simulink model "kopter_se_zavazim_state_feedback"  (R2024b)
(part 5 of 6)

0, 0, 0, 0, 0, 0, 0, 0, 0, 0, 0,                                                                                                                                                                                                                                                                                                                                                                                                                                                                                                                                                                                                                                                                                                                                                                                                                                                                                                                                                                                                                                                                                                                                                                                                  0,                                                                                                                                                                                                                                                                                                                                                                                                                                                                                                                                                                                                                                                                                                                                                                                                                                                                                                                                                                                                                                                                                                                                                                                                                                                                                                                                                                                                                                                                  0,                                                                                                                                                                                                                                                                                                                                                                                                                                                                                                                                                                                                                                                                                                                                                                                                                                                                                                                                                                                                                                                                                                                                                                                                        0, ((2*beta_dot_t*d*m*cos(alpha_t)*cos(beta_t) - alpha_dot_t*d*m*sin(alpha_t)*sin(beta_t))*(d^4*m^4*cos(beta_t)*sin(alpha_t)^4*sin(beta_t) - d^4*m^4*cos(beta_t)*sin(alpha_t)^2*sin(beta_t) - Ip*d^2*m^3*cos(beta_t)*sin(alpha_t)^2*sin(beta_t) - M*d^4*m^3*cos(beta_t)*sin(alpha_t)^2*sin(beta_t) + d^4*m^4*cos(alpha_t)^2*cos(beta_t)*sin(alpha_t)^2*sin(beta_t) + Ip*d^2*m^3*cos(alpha_t)^2*cos(beta_t)*sin(beta_t) + M*d^4*m^3*cos(alpha_t)^2*cos(beta_t)*sin(alpha_t)^2*sin(beta_t) + Ip*M*d^2*m^2*cos(alpha_t)^2*cos(beta_t)*sin(beta_t) - Ip*M*d^2*m^2*cos(beta_t)*sin(alpha_t)^2*sin(beta_t)))/(d^4*m^5*sin(alpha_t)^4 - Ip^2*m^3 - 3*Ip^2*M*m^2 - 3*Ip^2*M^2*m - d^4*m^5*sin(alpha_t)^2 - Ip^2*M^3 - Ip*d^2*m^4 + d^4*m^5*cos(beta_t)^2*sin(alpha_t)^2 - d^4*m^5*cos(beta_t)^2*sin(alpha_t)^4 + d^4*m^5*sin(alpha_t)^2*sin(beta_t)^2 - d^4*m^5*sin(alpha_t)^4*sin(beta_t)^2 - 3*M*d^4*m^4*sin(alpha_t)^2 + 2*M*d^4*m^4*sin(alpha_t)^4 - 3*Ip*M*d^2*m^3 - Ip*M^3*d^2*m - 3*M^2*d^4*m^3*sin(alpha_t)^2 - M^3*d^4*m^2*sin(alpha_t)^2 + M^2*d^4*m^3*sin(alpha_t)^4 - 3*Ip*M^2*d^2*m^2 + M^2*d^4*m^3*sin(alpha_t)^2*sin(beta_t)^2 - 2*Ip*M^2*d^2*m^2*sin(alpha_t)^2 + d^4*m^5*cos(alpha_t)^2*cos(beta_t)^2*sin(alpha_t)^2 - d^4*m^5*cos(alpha_t)^2*cos(beta_t)^4*sin(alpha_t)^2 + d^4*m^5*cos(alpha_t)^2*sin(alpha_t)^2*sin(beta_t)^2 - d^4*m^5*cos(alpha_t)^2*sin(alpha_t)^2*sin(beta_t)^4 + Ip*d^2*m^4*cos(alpha_t)^2*cos(beta_t)^2 + Ip*d^2*m^4*cos(alpha_t)^2*sin(beta_t)^2 + Ip*d^2*m^4*cos(beta_t)^2*sin(alpha_t)^2 + 2*M*d^4*m^4*cos(beta_t)^2*sin(alpha_t)^2 - M*d^4*m^4*cos(beta_t)^2*sin(alpha_t)^4 + Ip*d^2*m^4*sin(alpha_t)^2*sin(beta_t)^2 + 2*M*d^4*m^4*sin(alpha_t)^2*sin(beta_t)^2 - M*d^4*m^4*sin(alpha_t)^4*sin(beta_t)^2 - Ip*M*d^2*m^3*sin(alpha_t)^2 - Ip*M^3*d^2*m*sin(alpha_t)^2 + M^2*d^4*m^3*cos(beta_t)^2*sin(alpha_t)^2 + M^2*d^4*m^3*cos(alpha_t)^2*cos(beta_t)^2*sin(alpha_t)^2 + M^2*d^4*m^3*cos(alpha_t)^2*sin(alpha_t)^2*sin(beta_t)^2 + Ip*M^2*d^2*m^2*cos(alpha_t)^2*cos(beta_t)^2 + Ip*M^2*d^2*m^2*cos(alpha_t)^2*sin(beta_t)^2 + Ip*M^2*d^2*m^2*cos(beta_t)^2*sin(alpha_t)^2 + Ip*M^2*d^2*m^2*sin(alpha_t)^2*sin(beta_t)^2 - 2*d^4*m^5*cos(alpha_t)^2*cos(beta_t)^2*sin(alpha_t)^2*sin(beta_t)^2 + 2*M*d^4*m^4*cos(alpha_t)^2*cos(beta_t)^2*sin(alpha_t)^2 - M*d^4*m^4*cos(alpha_t)^2*cos(beta_t)^4*sin(alpha_t)^2 + 2*M*d^4*m^4*cos(alpha_t)^2*sin(alpha_t)^2*sin(beta_t)^2 - M*d^4*m^4*cos(alpha_t)^2*sin(alpha_t)^2*sin(beta_t)^4 + 2*Ip*M*d^2*m^3*cos(alpha_t)^2*cos(beta_t)^2 + 2*Ip*M*d^2*m^3*cos(alpha_t)^2*sin(beta_t)^2 + 2*Ip*M*d^2*m^3*cos(beta_t)^2*sin(alpha_t)^2 + 2*Ip*M*d^2*m^3*sin(alpha_t)^2*sin(beta_t)^2 - 2*M*d^4*m^4*cos(alpha_t)^2*cos(beta_t)^2*sin(alpha_t)^2*sin(beta_t)^2) - ((alpha_dot_t*d*m*cos(beta_t)*sin(alpha_t) + 2*beta_dot_t*d*m*cos(alpha_t)*sin(beta_t))*(Ip^2*M^2 + Ip^2*m^2 + d^4*m^4*sin(alpha_t)^2 - d^4*m^4*sin(alpha_t)^4 + Ip*d^2*m^3 + 2*Ip^2*M*m - d^4*m^4*cos(beta_t)^2*sin(alpha_t)^2 + d^4*m^4*cos(beta_t)^2*sin(alpha_t)^4 + 2*M*d^4*m^3*sin(alpha_t)^2 - M*d^4*m^3*sin(alpha_t)^4 + 2*Ip*M*d^2*m^2 + Ip*M^2*d^2*m + M^2*d^4*m^2*sin(alpha_t)^2 - d^4*m^4*cos(alpha_t)^2*sin(alpha_t)^2*sin(beta_t)^2 - Ip*d^2*m^3*cos(alpha_t)^2*sin(beta_t)^2 - Ip*d^2*m^3*cos(beta_t)^2*sin(alpha_t)^2 - M*d^4*m^3*cos(beta_t)^2*sin(alpha_t)^2 + Ip*M*d^2*m^2*sin(alpha_t)^2 + Ip*M^2*d^2*m*sin(alpha_t)^2 - M*d^4*m^3*cos(alpha_t)^2*sin(alpha_t)^2*sin(beta_t)^2 - Ip*M*d^2*m^2*cos(alpha_t)^2*sin(beta_t)^2 - Ip*M*d^2*m^2*cos(beta_t)^2*sin(alpha_t)^2))/(d^4*m^5*sin(alpha_t)^4 - Ip^2*m^3 - 3*Ip^2*M*m^2 - 3*Ip^2*M^2*m - d^4*m^5*sin(alpha_t)^2 - Ip^2*M^3 - Ip*d^2*m^4 + d^4*m^5*cos(beta_t)^2*sin(alpha_t)^2 - d^4*m^5*cos(beta_t)^2*sin(alpha_t)^4 + d^4*m^5*sin(alpha_t)^2*sin(beta_t)^2 - d^4*m^5*sin(alpha_t)^4*sin(beta_t)^2 - 3*M*d^4*m^4*sin(alpha_t)^2 + 2*M*d^4*m^4*sin(alpha_t)^4 - 3*Ip*M*d^2*m^3 - Ip*M^3*d^2*m - 3*M^2*d^4*m^3*sin(alpha_t)^2 - M^3*d^4*m^2*sin(alpha_t)^2 + M^2*d^4*m^3*sin(alpha_t)^4 - 3*Ip*M^2*d^2*m^2 + M^2*d^4*m^3*sin(alpha_t)^2*sin(beta_t)^2 - 2*Ip*M^2*d^2*m^2*sin(alpha_t)^2 + d^4*m^5*cos(alpha_t)^2*cos(beta_t)^2*sin(alpha_t)^2 - d^4*m^5*cos(alpha_t)^2*cos(beta_t)^4*sin(alpha_t)^2 + d^4*m^5*cos(alpha_t)^2*sin(alpha_t)^2*sin(beta_t)^2 - d^4*m^5*cos(alpha_t)^2*sin(alpha_t)^2*sin(beta_t)^4 + Ip*d^2*m^4*cos(alpha_t)^2*cos(beta_t)^2 + Ip*d^2*m^4*cos(alpha_t)^2*sin(beta_t)^2 + Ip*d^2*m^4*cos(beta_t)^2*sin(alpha_t)^2 + 2*M*d^4*m^4*cos(beta_t)^2*sin(alpha_t)^2 - M*d^4*m^4*cos(beta_t)^2*sin(alpha_t)^4 + Ip*d^2*m^4*sin(alpha_t)^2*sin(beta_t)^2 + 2*M*d^4*m^4*sin(alpha_t)^2*sin(beta_t)^2 - M*d^4*m^4*sin(alpha_t)^4*sin(beta_t)^2 - Ip*M*d^2*m^3*sin(alpha_t)^2 - Ip*M^3*d^2*m*sin(alpha_t)^2 + M^2*d^4*m^3*cos(beta_t)^2*sin(alpha_t)^2 + M^2*d^4*m^3*cos(alpha_t)^2*cos(beta_t)^2*sin(alpha_t)^2 + M^2*d^4*m^3*cos(alpha_t)^2*sin(alpha_t)^2*sin(beta_t)^2 + Ip*M^2*d^2*m^2*cos(alpha_t)^2*cos(beta_t)^2 + Ip*M^2*d^2*m^2*cos(alpha_t)^2*sin(beta_t)^2 + Ip*M^2*d^2*m^2*cos(beta_t)^2*sin(alpha_t)^2 + Ip*M^2*d^2*m^2*sin(alpha_t)^2*sin(beta_t)^2 - 2*d^4*m^5*cos(alpha_t)^2*cos(beta_t)^2*sin(alpha_t)^2*sin(beta_t)^2 + 2*M*d^4*m^4*cos(alpha_t)^2*cos(beta_t)^2*sin(alpha_t)^2 - M*d^4*m^4*cos(alpha_t)^2*cos(beta_t)^4*sin(alpha_t)^2 + 2*M*d^4*m^4*cos(alpha_t)^2*sin(alpha_t)^2*sin(beta_t)^2 - M*d^4*m^4*cos(alpha_t)^2*sin(alpha_t)^2*sin(beta_t)^4 + 2*Ip*M*d^2*m^3*cos(alpha_t)^2*cos(beta_t)^2 + 2*Ip*M*d^2*m^3*cos(alpha_t)^2*sin(beta_t)^2 + 2*Ip*M*d^2*m^3*cos(beta_t)^2*sin(alpha_t)^2 + 2*Ip*M*d^2*m^3*sin(alpha_t)^2*sin(beta_t)^2 - 2*M*d^4*m^4*cos(alpha_t)^2*cos(beta_t)^2*sin(alpha_t)^2*sin(beta_t)^2) - (alpha_dot_t*d*m*cos(alpha_t)*cos(beta_t)*(d^2*m*cos(alpha_t)*cos(beta_t)^2*sin(alpha_t) - d^2*m*cos(alpha_t)*sin(alpha_t) + d^2*m*cos(alpha_t)*sin(alpha_t)*sin(beta_t)^2))/(- d^2*m^2*cos(alpha_t)^2*cos(beta_t)^2 - d^2*m^2*cos(alpha_t)^2*sin(beta_t)^2 - d^2*m^2*sin(alpha_t)^2 + d^2*m^2 + M*d^2*m + Ip*m + Ip*M) - (alpha_dot_t*d^3*m^3*cos(alpha_t)^2*cos(beta_t)*sin(alpha_t))/(Ip*M^2 + Ip*m^2 + d^2*m^3 - d^2*m^3*sin(alpha_t)^2 + 2*M*d^2*m^2 + M^2*d^2*m + 2*Ip*M*m - d^2*m^3*cos(alpha_t)^2*cos(beta_t)^2 - d^2*m^3*cos(alpha_t)^2*sin(beta_t)^2 - M*d^2*m^2*sin(alpha_t)^2 - M*d^2*m^2*cos(alpha_t)^2*cos(beta_t)^2 - M*d^2*m^2*cos(alpha_t)^2*sin(beta_t)^2) - (beta_dot_t*d*m*sin(alpha_t)*sin(beta_t)*(2*d^2*m*cos(alpha_t)*cos(beta_t)^2*sin(alpha_t) + 2*d^2*m*cos(alpha_t)*sin(alpha_t)*sin(beta_t)^2))/(- d^2*m^2*cos(beta_t)^2*sin(alpha_t)^2 - d^2*m^2*sin(alpha_t)^2*sin(beta_t)^2 + d^2*m^2*sin(alpha_t)^2 + M*d^2*m*sin(alpha_t)^2 + Ip*m + Ip*M), - (beta_dot_t*d*m*cos(alpha_t)*cos(beta_t)*(m*cos(alpha_t)*sin(alpha_t)*d^2*cos(beta_t)^2 + m*cos(alpha_t)*sin(alpha_t)*d^2*sin(beta_t)^2))/(- d^2*m^2*cos(alpha_t)^2*cos(beta_t)^2 - d^2*m^2*cos(alpha_t)^2*sin(beta_t)^2 - d^2*m^2*sin(alpha_t)^2 + d^2*m^2 + M*d^2*m + Ip*m + Ip*M) - (beta_dot_t*d*m*sin(alpha_t)*sin(beta_t)*(d^4*m^4*cos(beta_t)*sin(alpha_t)^4*sin(beta_t) - d^4*m^4*cos(beta_t)*sin(alpha_t)^2*sin(beta_t) - Ip*d^2*m^3*cos(beta_t)*sin(alpha_t)^2*sin(beta_t) - M*d^4*m^3*cos(beta_t)*sin(alpha_t)^2*sin(beta_t) + d^4*m^4*cos(alpha_t)^2*cos(beta_t)*sin(alpha_t)^2*sin(beta_t) + Ip*d^2*m^3*cos(alpha_t)^2*cos(beta_t)*sin(beta_t) + M*d^4*m^3*cos(alpha_t)^2*cos(beta_t)*sin(alpha_t)^2*sin(beta_t) + Ip*M*d^2*m^2*cos(alpha_t)^2*cos(beta_t)*sin(beta_t) - Ip*M*d^2*m^2*cos(beta_t)*sin(alpha_t)^2*sin(beta_t)))/(d^4*m^5*sin(alpha_t)^4 - Ip^2*m^3 - 3*Ip^2*M*m^2 - 3*Ip^2*M^2*m - d^4*m^5*sin(alpha_t)^2 - Ip^2*M^3 - Ip*d^2*m^4 + d^4*m^5*cos(beta_t)^2*sin(alpha_t)^2 - d^4*m^5*cos(beta_t)^2*sin(alpha_t)^4 + d^4*m^5*sin(alpha_t)^2*sin(beta_t)^2 - d^4*m^5*sin(alpha_t)^4*sin(beta_t)^2 - 3*M*d^4*m^4*sin(alpha_t)^2 + 2*M*d^4*m^4*sin(alpha_t)^4 - 3*Ip*M*d^2*m^3 - Ip*M^3*d^2*m - 3*M^2*d^4*m^3*sin(alpha_t)^2 - M^3*d^4*m^2*sin(alpha_t)^2 + M^2*d^4*m^3*sin(alpha_t)^4 - 3*Ip*M^2*d^2*m^2 + M^2*d^4*m^3*sin(alpha_t)^2*sin(beta_t)^2 - 2*Ip*M^2*d^2*m^2*sin(alpha_t)^2 + d^4*m^5*cos(alpha_t)^2*cos(beta_t)^2*sin(alpha_t)^2 - d^4*m^5*cos(alpha_t)^2*cos(beta_t)^4*sin(alpha_t)^2 + d^4*m^5*cos(alpha_t)^2*sin(alpha_t)^2*sin(beta_t)^2 - d^4*m^5*cos(alpha_t)^2*sin(alpha_t)^2*sin(beta_t)^4 + Ip*d^2*m^4*cos(alpha_t)^2*cos(beta_t)^2 + Ip*d^2*m^4*cos(alpha_t)^2*sin(beta_t)^2 + Ip*d^2*m^4*cos(beta_t)^2*sin(alpha_t)^2 + 2*M*d^4*m^4*cos(beta_t)^2*sin(alpha_t)^2 - M*d^4*m^4*cos(beta_t)^2*sin(alpha_t)^4 + Ip*d^2*m^4*sin(alpha_t)^2*sin(beta_t)^2 + 2*M*d^4*m^4*sin(alpha_t)^2*sin(beta_t)^2 - M*d^4*m^4*sin(alpha_t)^4*sin(beta_t)^2 - Ip*M*d^2*m^3*sin(alpha_t)^2 - Ip*M^3*d^2*m*sin(alpha_t)^2 + M^2*d^4*m^3*cos(beta_t)^2*sin(alpha_t)^2 + M^2*d^4*m^3*cos(alpha_t)^2*cos(beta_t)^2*sin(alpha_t)^2 + M^2*d^4*m^3*cos(alpha_t)^2*sin(alpha_t)^2*sin(beta_t)^2 + Ip*M^2*d^2*m^2*cos(alpha_t)^2*cos(beta_t)^2 + Ip*M^2*d^2*m^2*cos(alpha_t)^2*sin(beta_t)^2 + Ip*M^2*d^2*m^2*cos(beta_t)^2*sin(alpha_t)^2 + Ip*M^2*d^2*m^2*sin(alpha_t)^2*sin(beta_t)^2 - 2*d^4*m^5*cos(alpha_t)^2*cos(beta_t)^2*sin(alpha_t)^2*sin(beta_t)^2 + 2*M*d^4*m^4*cos(alpha_t)^2*cos(beta_t)^2*sin(alpha_t)^2 - M*d^4*m^4*cos(alpha_t)^2*cos(beta_t)^4*sin(alpha_t)^2 + 2*M*d^4*m^4*cos(alpha_t)^2*sin(alpha_t)^2*sin(beta_t)^2 - M*d^4*m^4*cos(alpha_t)^2*sin(alpha_t)^2*sin(beta_t)^4 + 2*Ip*M*d^2*m^3*cos(alpha_t)^2*cos(beta_t)^2 + 2*Ip*M*d^2*m^3*cos(alpha_t)^2*sin(beta_t)^2 + 2*Ip*M*d^2*m^3*cos(beta_t)^2*sin(alpha_t)^2 + 2*Ip*M*d^2*m^3*sin(alpha_t)^2*sin(beta_t)^2 - 2*M*d^4*m^4*cos(alpha_t)^2*cos(beta_t)^2*sin(alpha_t)^2*sin(beta_t)^2) - (beta_dot_t*d*m*cos(beta_t)*sin(alpha_t)*(Ip^2*M^2 + Ip^2*m^2 + d^4*m^4*sin(alpha_t)^2 - d^4*m^4*sin(alpha_t)^4 + Ip*d^2*m^3 + 2*Ip^2*M*m - d^4*m^4*cos(beta_t)^2*sin(alpha_t)^2 + d^4*m^4*cos(beta_t)^2*sin(alpha_t)^4 + 2*M*d^4*m^3*sin(alpha_t)^2 - M*d^4*m^3*sin(alpha_t)^4 + 2*Ip*M*d^2*m^2 + Ip*M^2*d^2*m + M^2*d^4*m^2*sin(alpha_t)^2 - d^4*m^4*cos(alpha_t)^2*sin(alpha_t)^2*sin(beta_t)^2 - Ip*d^2*m^3*cos(alpha_t)^2*sin(beta_t)^2 - Ip*d^2*m^3*cos(beta_t)^2*sin(alpha_t)^2 - M*d^4*m^3*cos(beta_t)^2*sin(alpha_t)^2 + Ip*M*d^2*m^2*sin(alpha_t)^2 + Ip*M^2*d^2*m*sin(alpha_t)^2 - M*d^4*m^3*cos(alpha_t)^2*sin(alpha_t)^2*sin(beta_t)^2 - Ip*M*d^2*m^2*cos(alpha_t)^2*sin(beta_t)^2 - Ip*M*d^2*m^2*cos(beta_t)^2*sin(alpha_t)^2))/(d^4*m^5*sin(alpha_t)^4 - Ip^2*m^3 - 3*Ip^2*M*m^2 - 3*Ip^2*M^2*m - d^4*m^5*sin(alpha_t)^2 - Ip^2*M^3 - Ip*d^2*m^4 + d^4*m^5*cos(beta_t)^2*sin(alpha_t)^2 - d^4*m^5*cos(beta_t)^2*sin(alpha_t)^4 + d^4*m^5*sin(alpha_t)^2*sin(beta_t)^2 - d^4*m^5*sin(alpha_t)^4*sin(beta_t)^2 - 3*M*d^4*m^4*sin(alpha_t)^2 + 2*M*d^4*m^4*sin(alpha_t)^4 - 3*Ip*M*d^2*m^3 - Ip*M^3*d^2*m - 3*M^2*d^4*m^3*sin(alpha_t)^2 - M^3*d^4*m^2*sin(alpha_t)^2 + M^2*d^4*m^3*sin(alpha_t)^4 - 3*Ip*M^2*d^2*m^2 + M^2*d^4*m^3*sin(alpha_t)^2*sin(beta_t)^2 - 2*Ip*M^2*d^2*m^2*sin(alpha_t)^2 + d^4*m^5*cos(alpha_t)^2*cos(beta_t)^2*sin(alpha_t)^2 - d^4*m^5*cos(alpha_t)^2*cos(beta_t)^4*sin(alpha_t)^2 + d^4*m^5*cos(alpha_t)^2*sin(alpha_t)^2*sin(beta_t)^2 - d^4*m^5*cos(alpha_t)^2*sin(alpha_t)^2*sin(beta_t)^4 + Ip*d^2*m^4*cos(alpha_t)^2*cos(beta_t)^2 + Ip*d^2*m^4*cos(alpha_t)^2*sin(beta_t)^2 + Ip*d^2*m^4*cos(beta_t)^2*sin(alpha_t)^2 + 2*M*d^4*m^4*cos(beta_t)^2*sin(alpha_t)^2 - M*d^4*m^4*cos(beta_t)^2*sin(alpha_t)^4 + Ip*d^2*m^4*sin(alpha_t)^2*sin(beta_t)^2 + 2*M*d^4*m^4*sin(alpha_t)^2*sin(beta_t)^2 - M*d^4*m^4*sin(alpha_t)^4*sin(beta_t)^2 - Ip*M*d^2*m^3*sin(alpha_t)^2 - Ip*M^3*d^2*m*sin(alpha_t)^2 + M^2*d^4*m^3*cos(beta_t)^2*sin(alpha_t)^2 + M^2*d^4*m^3*cos(alpha_t)^2*cos(beta_t)^2*sin(alpha_t)^2 + M^2*d^4*m^3*cos(alpha_t)^2*sin(alpha_t)^2*sin(beta_t)^2 + Ip*M^2*d^2*m^2*cos(alpha_t)^2*cos(beta_t)^2 + Ip*M^2*d^2*m^2*cos(alpha_t)^2*sin(beta_t)^2 + Ip*M^2*d^2*m^2*cos(beta_t)^2*sin(alpha_t)^2 + Ip*M^2*d^2*m^2*sin(alpha_t)^2*sin(beta_t)^2 - 2*d^4*m^5*cos(alpha_t)^2*cos(beta_t)^2*sin(alpha_t)^2*sin(beta_t)^2 + 2*M*d^4*m^4*cos(alpha_t)^2*cos(beta_t)^2*sin(alpha_t)^2 - M*d^4*m^4*cos(alpha_t)^2*cos(beta_t)^4*sin(alpha_t)^2 + 2*M*d^4*m^4*cos(alpha_t)^2*sin(alpha_t)^2*sin(beta_t)^2 - M*d^4*m^4*cos(alpha_t)^2*sin(alpha_t)^2*sin(beta_t)^4 + 2*Ip*M*d^2*m^3*cos(alpha_t)^2*cos(beta_t)^2 + 2*Ip*M*d^2*m^3*cos(alpha_t)^2*sin(beta_t)^2 + 2*Ip*M*d^2*m^3*cos(beta_t)^2*sin(alpha_t)^2 + 2*Ip*M*d^2*m^3*sin(alpha_t)^2*sin(beta_t)^2 - 2*M*d^4*m^4*cos(alpha_t)^2*cos(beta_t)^2*sin(alpha_t)^2*sin(beta_t)^2);
0, 0, 0, 0, 0, 0, 0, 0, 0, 0, 0,                                                                                                                                                                                                                                                                                                                                                                                                                                                                                                                                                                                                                                                                                                                                                                                                                                                                                                                                                                                                                                                                                                                                                                                                  0,                                                                                                                                                                                                                                                                                                                                                                                                                                                                                                                                                                                                                                                                                                                                                                                                                                                                                                                                                                                                                                                                                                                                                                                                                                                                                                                                                                                                                                                                  0,                                                                                                                                                                                                                                                                                                                                                                                                                                                                                                                                                                                                                                                                                                                                                                                                                                                                                                                                                                                                                                                                                                                                                                                                        0, ((2*beta_dot_t*d*m*cos(alpha_t)*cos(beta_t) - alpha_dot_t*d*m*sin(alpha_t)*sin(beta_t))*(Ip^2*M^2 + Ip^2*m^2 + d^4*m^4*sin(alpha_t)^2 - d^4*m^4*sin(alpha_t)^4 + Ip*d^2*m^3 + 2*Ip^2*M*m - d^4*m^4*sin(alpha_t)^2*sin(beta_t)^2 + d^4*m^4*sin(alpha_t)^4*sin(beta_t)^2 + 2*M*d^4*m^3*sin(alpha_t)^2 - M*d^4*m^3*sin(alpha_t)^4 + 2*Ip*M*d^2*m^2 + Ip*M^2*d^2*m + M^2*d^4*m^2*sin(alpha_t)^2 - d^4*m^4*cos(alpha_t)^2*cos(beta_t)^2*sin(alpha_t)^2 - Ip*d^2*m^3*cos(alpha_t)^2*cos(beta_t)^2 - Ip*d^2*m^3*sin(alpha_t)^2*sin(beta_t)^2 - M*d^4*m^3*sin(alpha_t)^2*sin(beta_t)^2 + Ip*M*d^2*m^2*sin(alpha_t)^2 + Ip*M^2*d^2*m*sin(alpha_t)^2 - M*d^4*m^3*cos(alpha_t)^2*cos(beta_t)^2*sin(alpha_t)^2 - Ip*M*d^2*m^2*cos(alpha_t)^2*cos(beta_t)^2 - Ip*M*d^2*m^2*sin(alpha_t)^2*sin(beta_t)^2))/(d^4*m^5*sin(alpha_t)^4 - Ip^2*m^3 - 3*Ip^2*M*m^2 - 3*Ip^2*M^2*m - d^4*m^5*sin(alpha_t)^2 - Ip^2*M^3 - Ip*d^2*m^4 + d^4*m^5*cos(beta_t)^2*sin(alpha_t)^2 - d^4*m^5*cos(beta_t)^2*sin(alpha_t)^4 + d^4*m^5*sin(alpha_t)^2*sin(beta_t)^2 - d^4*m^5*sin(alpha_t)^4*sin(beta_t)^2 - 3*M*d^4*m^4*sin(alpha_t)^2 + 2*M*d^4*m^4*sin(alpha_t)^4 - 3*Ip*M*d^2*m^3 - Ip*M^3*d^2*m - 3*M^2*d^4*m^3*sin(alpha_t)^2 - M^3*d^4*m^2*sin(alpha_t)^2 + M^2*d^4*m^3*sin(alpha_t)^4 - 3*Ip*M^2*d^2*m^2 + M^2*d^4*m^3*sin(alpha_t)^2*sin(beta_t)^2 - 2*Ip*M^2*d^2*m^2*sin(alpha_t)^2 + d^4*m^5*cos(alpha_t)^2*cos(beta_t)^2*sin(alpha_t)^2 - d^4*m^5*cos(alpha_t)^2*cos(beta_t)^4*sin(alpha_t)^2 + d^4*m^5*cos(alpha_t)^2*sin(alpha_t)^2*sin(beta_t)^2 - d^4*m^5*cos(alpha_t)^2*sin(alpha_t)^2*sin(beta_t)^4 + Ip*d^2*m^4*cos(alpha_t)^2*cos(beta_t)^2 + Ip*d^2*m^4*cos(alpha_t)^2*sin(beta_t)^2 + Ip*d^2*m^4*cos(beta_t)^2*sin(alpha_t)^2 + 2*M*d^4*m^4*cos(beta_t)^2*sin(alpha_t)^2 - M*d^4*m^4*cos(beta_t)^2*sin(alpha_t)^4 + Ip*d^2*m^4*sin(alpha_t)^2*sin(beta_t)^2 + 2*M*d^4*m^4*sin(alpha_t)^2*sin(beta_t)^2 - M*d^4*m^4*sin(alpha_t)^4*sin(beta_t)^2 - Ip*M*d^2*m^3*sin(alpha_t)^2 - Ip*M^3*d^2*m*sin(alpha_t)^2 + M^2*d^4*m^3*cos(beta_t)^2*sin(alpha_t)^2 + M^2*d^4*m^3*cos(alpha_t)^2*cos(beta_t)^2*sin(alpha_t)^2 + M^2*d^4*m^3*cos(alpha_t)^2*sin(alpha_t)^2*sin(beta_t)^2 + Ip*M^2*d^2*m^2*cos(alpha_t)^2*cos(beta_t)^2 + Ip*M^2*d^2*m^2*cos(alpha_t)^2*sin(beta_t)^2 + Ip*M^2*d^2*m^2*cos(beta_t)^2*sin(alpha_t)^2 + Ip*M^2*d^2*m^2*sin(alpha_t)^2*sin(beta_t)^2 - 2*d^4*m^5*cos(alpha_t)^2*cos(beta_t)^2*sin(alpha_t)^2*sin(beta_t)^2 + 2*M*d^4*m^4*cos(alpha_t)^2*cos(beta_t)^2*sin(alpha_t)^2 - M*d^4*m^4*cos(alpha_t)^2*cos(beta_t)^4*sin(alpha_t)^2 + 2*M*d^4*m^4*cos(alpha_t)^2*sin(alpha_t)^2*sin(beta_t)^2 - M*d^4*m^4*cos(alpha_t)^2*sin(alpha_t)^2*sin(beta_t)^4 + 2*Ip*M*d^2*m^3*cos(alpha_t)^2*cos(beta_t)^2 + 2*Ip*M*d^2*m^3*cos(alpha_t)^2*sin(beta_t)^2 + 2*Ip*M*d^2*m^3*cos(beta_t)^2*sin(alpha_t)^2 + 2*Ip*M*d^2*m^3*sin(alpha_t)^2*sin(beta_t)^2 - 2*M*d^4*m^4*cos(alpha_t)^2*cos(beta_t)^2*sin(alpha_t)^2*sin(beta_t)^2) - ((alpha_dot_t*d*m*cos(beta_t)*sin(alpha_t) + 2*beta_dot_t*d*m*cos(alpha_t)*sin(beta_t))*(d^4*m^4*cos(beta_t)*sin(alpha_t)^4*sin(beta_t) - d^4*m^4*cos(beta_t)*sin(alpha_t)^2*sin(beta_t) - Ip*d^2*m^3*cos(beta_t)*sin(alpha_t)^2*sin(beta_t) - M*d^4*m^3*cos(beta_t)*sin(alpha_t)^2*sin(beta_t) + d^4*m^4*cos(alpha_t)^2*cos(beta_t)*sin(alpha_t)^2*sin(beta_t) + Ip*d^2*m^3*cos(alpha_t)^2*cos(beta_t)*sin(beta_t) + M*d^4*m^3*cos(alpha_t)^2*cos(beta_t)*sin(alpha_t)^2*sin(beta_t) + Ip*M*d^2*m^2*cos(alpha_t)^2*cos(beta_t)*sin(beta_t) - Ip*M*d^2*m^2*cos(beta_t)*sin(alpha_t)^2*sin(beta_t)))/(d^4*m^5*sin(alpha_t)^4 - Ip^2*m^3 - 3*Ip^2*M*m^2 - 3*Ip^2*M^2*m - d^4*m^5*sin(alpha_t)^2 - Ip^2*M^3 - Ip*d^2*m^4 + d^4*m^5*cos(beta_t)^2*sin(alpha_t)^2 - d^4*m^5*cos(beta_t)^2*sin(alpha_t)^4 + d^4*m^5*sin(alpha_t)^2*sin(beta_t)^2 - d^4*m^5*sin(alpha_t)^4*sin(beta_t)^2 - 3*M*d^4*m^4*sin(alpha_t)^2 + 2*M*d^4*m^4*sin(alpha_t)^4 - 3*Ip*M*d^2*m^3 - Ip*M^3*d^2*m - 3*M^2*d^4*m^3*sin(alpha_t)^2 - M^3*d^4*m^2*sin(alpha_t)^2 + M^2*d^4*m^3*sin(alpha_t)^4 - 3*Ip*M^2*d^2*m^2 + M^2*d^4*m^3*sin(alpha_t)^2*sin(beta_t)^2 - 2*Ip*M^2*d^2*m^2*sin(alpha_t)^2 + d^4*m^5*cos(alpha_t)^2*cos(beta_t)^2*sin(alpha_t)^2 - d^4*m^5*cos(alpha_t)^2*cos(beta_t)^4*sin(alpha_t)^2 + d^4*m^5*cos(alpha_t)^2*sin(alpha_t)^2*sin(beta_t)^2 - d^4*m^5*cos(alpha_t)^2*sin(alpha_t)^2*sin(beta_t)^4 + Ip*d^2*m^4*cos(alpha_t)^2*cos(beta_t)^2 + Ip*d^2*m^4*cos(alpha_t)^2*sin(beta_t)^2 + Ip*d^2*m^4*cos(beta_t)^2*sin(alpha_t)^2 + 2*M*d^4*m^4*cos(beta_t)^2*sin(alpha_t)^2 - M*d^4*m^4*cos(beta_t)^2*sin(alpha_t)^4 + Ip*d^2*m^4*sin(alpha_t)^2*sin(beta_t)^2 + 2*M*d^4*m^4*sin(alpha_t)^2*sin(beta_t)^2 - M*d^4*m^4*sin(alpha_t)^4*sin(beta_t)^2 - Ip*M*d^2*m^3*sin(alpha_t)^2 - Ip*M^3*d^2*m*sin(alpha_t)^2 + M^2*d^4*m^3*cos(beta_t)^2*sin(alpha_t)^2 + M^2*d^4*m^3*cos(alpha_t)^2*cos(beta_t)^2*sin(alpha_t)^2 + M^2*d^4*m^3*cos(alpha_t)^2*sin(alpha_t)^2*sin(beta_t)^2 + Ip*M^2*d^2*m^2*cos(alpha_t)^2*cos(beta_t)^2 + Ip*M^2*d^2*m^2*cos(alpha_t)^2*sin(beta_t)^2 + Ip*M^2*d^2*m^2*cos(beta_t)^2*sin(alpha_t)^2 + Ip*M^2*d^2*m^2*sin(alpha_t)^2*sin(beta_t)^2 - 2*d^4*m^5*cos(alpha_t)^2*cos(beta_t)^2*sin(alpha_t)^2*sin(beta_t)^2 + 2*M*d^4*m^4*cos(alpha_t)^2*cos(beta_t)^2*sin(alpha_t)^2 - M*d^4*m^4*cos(alpha_t)^2*cos(beta_t)^4*sin(alpha_t)^2 + 2*M*d^4*m^4*cos(alpha_t)^2*sin(alpha_t)^2*sin(beta_t)^2 - M*d^4*m^4*cos(alpha_t)^2*sin(alpha_t)^2*sin(beta_t)^4 + 2*Ip*M*d^2*m^3*cos(alpha_t)^2*cos(beta_t)^2 + 2*Ip*M*d^2*m^3*cos(alpha_t)^2*sin(beta_t)^2 + 2*Ip*M*d^2*m^3*cos(beta_t)^2*sin(alpha_t)^2 + 2*Ip*M*d^2*m^3*sin(alpha_t)^2*sin(beta_t)^2 - 2*M*d^4*m^4*cos(alpha_t)^2*cos(beta_t)^2*sin(alpha_t)^2*sin(beta_t)^2) - (alpha_dot_t*d*m*cos(alpha_t)*sin(beta_t)*(d^2*m*cos(alpha_t)*cos(beta_t)^2*sin(alpha_t) - d^2*m*cos(alpha_t)*sin(alpha_t) + d^2*m*cos(alpha_t)*sin(alpha_t)*sin(beta_t)^2))/(- d^2*m^2*cos(alpha_t)^2*cos(beta_t)^2 - d^2*m^2*cos(alpha_t)^2*sin(beta_t)^2 - d^2*m^2*sin(alpha_t)^2 + d^2*m^2 + M*d^2*m + Ip*m + Ip*M) - (alpha_dot_t*d^3*m^3*cos(alpha_t)^2*sin(alpha_t)*sin(beta_t))/(Ip*M^2 + Ip*m^2 + d^2*m^3 - d^2*m^3*sin(alpha_t)^2 + 2*M*d^2*m^2 + M^2*d^2*m + 2*Ip*M*m - d^2*m^3*cos(alpha_t)^2*cos(beta_t)^2 - d^2*m^3*cos(alpha_t)^2*sin(beta_t)^2 - M*d^2*m^2*sin(alpha_t)^2 - M*d^2*m^2*cos(alpha_t)^2*cos(beta_t)^2 - M*d^2*m^2*cos(alpha_t)^2*sin(beta_t)^2) + (beta_dot_t*d*m*cos(beta_t)*sin(alpha_t)*(2*d^2*m*cos(alpha_t)*cos(beta_t)^2*sin(alpha_t) + 2*d^2*m*cos(alpha_t)*sin(alpha_t)*sin(beta_t)^2))/(- d^2*m^2*cos(beta_t)^2*sin(alpha_t)^2 - d^2*m^2*sin(alpha_t)^2*sin(beta_t)^2 + d^2*m^2*sin(alpha_t)^2 + M*d^2*m*sin(alpha_t)^2 + Ip*m + Ip*M), - (beta_dot_t*d*m*cos(alpha_t)*sin(beta_t)*(m*cos(alpha_t)*sin(alpha_t)*d^2*cos(beta_t)^2 + m*cos(alpha_t)*sin(alpha_t)*d^2*sin(beta_t)^2))/(- d^2*m^2*cos(alpha_t)^2*cos(beta_t)^2 - d^2*m^2*cos(alpha_t)^2*sin(beta_t)^2 - d^2*m^2*sin(alpha_t)^2 + d^2*m^2 + M*d^2*m + Ip*m + Ip*M) - (beta_dot_t*d*m*cos(beta_t)*sin(alpha_t)*(d^4*m^4*cos(beta_t)*sin(alpha_t)^4*sin(beta_t) - d^4*m^4*cos(beta_t)*sin(alpha_t)^2*sin(beta_t) - Ip*d^2*m^3*cos(beta_t)*sin(alpha_t)^2*sin(beta_t) - M*d^4*m^3*cos(beta_t)*sin(alpha_t)^2*sin(beta_t) + d^4*m^4*cos(alpha_t)^2*cos(beta_t)*sin(alpha_t)^2*sin(beta_t) + Ip*d^2*m^3*cos(alpha_t)^2*cos(beta_t)*sin(beta_t) + M*d^4*m^3*cos(alpha_t)^2*cos(beta_t)*sin(alpha_t)^2*sin(beta_t) + Ip*M*d^2*m^2*cos(alpha_t)^2*cos(beta_t)*sin(beta_t) - Ip*M*d^2*m^2*cos(beta_t)*sin(alpha_t)^2*sin(beta_t)))/(d^4*m^5*sin(alpha_t)^4 - Ip^2*m^3 - 3*Ip^2*M*m^2 - 3*Ip^2*M^2*m - d^4*m^5*sin(alpha_t)^2 - Ip^2*M^3 - Ip*d^2*m^4 + d^4*m^5*cos(beta_t)^2*sin(alpha_t)^2 - d^4*m^5*cos(beta_t)^2*sin(alpha_t)^4 + d^4*m^5*sin(alpha_t)^2*sin(beta_t)^2 - d^4*m^5*sin(alpha_t)^4*sin(beta_t)^2 - 3*M*d^4*m^4*sin(alpha_t)^2 + 2*M*d^4*m^4*sin(alpha_t)^4 - 3*Ip*M*d^2*m^3 - Ip*M^3*d^2*m - 3*M^2*d^4*m^3*sin(alpha_t)^2 - M^3*d^4*m^2*sin(alpha_t)^2 + M^2*d^4*m^3*sin(alpha_t)^4 - 3*Ip*M^2*d^2*m^2 + M^2*d^4*m^3*sin(alpha_t)^2*sin(beta_t)^2 - 2*Ip*M^2*d^2*m^2*sin(alpha_t)^2 + d^4*m^5*cos(alpha_t)^2*cos(beta_t)^2*sin(alpha_t)^2 - d^4*m^5*cos(alpha_t)^2*cos(beta_t)^4*sin(alpha_t)^2 + d^4*m^5*cos(alpha_t)^2*sin(alpha_t)^2*sin(beta_t)^2 - d^4*m^5*cos(alpha_t)^2*sin(alpha_t)^2*sin(beta_t)^4 + Ip*d^2*m^4*cos(alpha_t)^2*cos(beta_t)^2 + Ip*d^2*m^4*cos(alpha_t)^2*sin(beta_t)^2 + Ip*d^2*m^4*cos(beta_t)^2*sin(alpha_t)^2 + 2*M*d^4*m^4*cos(beta_t)^2*sin(alpha_t)^2 - M*d^4*m^4*cos(beta_t)^2*sin(alpha_t)^4 + Ip*d^2*m^4*sin(alpha_t)^2*sin(beta_t)^2 + 2*M*d^4*m^4*sin(alpha_t)^2*sin(beta_t)^2 - M*d^4*m^4*sin(alpha_t)^4*sin(beta_t)^2 - Ip*M*d^2*m^3*sin(alpha_t)^2 - Ip*M^3*d^2*m*sin(alpha_t)^2 + M^2*d^4*m^3*cos(beta_t)^2*sin(alpha_t)^2 + M^2*d^4*m^3*cos(alpha_t)^2*cos(beta_t)^2*sin(alpha_t)^2 + M^2*d^4*m^3*cos(alpha_t)^2*sin(alpha_t)^2*sin(beta_t)^2 + Ip*M^2*d^2*m^2*cos(alpha_t)^2*cos(beta_t)^2 + Ip*M^2*d^2*m^2*cos(alpha_t)^2*sin(beta_t)^2 + Ip*M^2*d^2*m^2*cos(beta_t)^2*sin(alpha_t)^2 + Ip*M^2*d^2*m^2*sin(alpha_t)^2*sin(beta_t)^2 - 2*d^4*m^5*cos(alpha_t)^2*cos(beta_t)^2*sin(alpha_t)^2*sin(beta_t)^2 + 2*M*d^4*m^4*cos(alpha_t)^2*cos(beta_t)^2*sin(alpha_t)^2 - M*d^4*m^4*cos(alpha_t)^2*cos(beta_t)^4*sin(alpha_t)^2 + 2*M*d^4*m^4*cos(alpha_t)^2*sin(alpha_t)^2*sin(beta_t)^2 - M*d^4*m^4*cos(alpha_t)^2*sin(alpha_t)^2*sin(beta_t)^4 + 2*Ip*M*d^2*m^3*cos(alpha_t)^2*cos(beta_t)^2 + 2*Ip*M*d^2*m^3*cos(alpha_t)^2*sin(beta_t)^2 + 2*Ip*M*d^2*m^3*cos(beta_t)^2*sin(alpha_t)^2 + 2*Ip*M*d^2*m^3*sin(alpha_t)^2*sin(beta_t)^2 - 2*M*d^4*m^4*cos(alpha_t)^2*cos(beta_t)^2*sin(alpha_t)^2*sin(beta_t)^2) - (beta_dot_t*d*m*sin(alpha_t)*sin(beta_t)*(Ip^2*M^2 + Ip^2*m^2 + d^4*m^4*sin(alpha_t)^2 - d^4*m^4*sin(alpha_t)^4 + Ip*d^2*m^3 + 2*Ip^2*M*m - d^4*m^4*sin(alpha_t)^2*sin(beta_t)^2 + d^4*m^4*sin(alpha_t)^4*sin(beta_t)^2 + 2*M*d^4*m^3*sin(alpha_t)^2 - M*d^4*m^3*sin(alpha_t)^4 + 2*Ip*M*d^2*m^2 + Ip*M^2*d^2*m + M^2*d^4*m^2*sin(alpha_t)^2 - d^4*m^4*cos(alpha_t)^2*cos(beta_t)^2*sin(alpha_t)^2 - Ip*d^2*m^3*cos(alpha_t)^2*cos(beta_t)^2 - Ip*d^2*m^3*sin(alpha_t)^2*sin(beta_t)^2 - M*d^4*m^3*sin(alpha_t)^2*sin(beta_t)^2 + Ip*M*d^2*m^2*sin(alpha_t)^2 + Ip*M^2*d^2*m*sin(alpha_t)^2 - M*d^4*m^3*cos(alpha_t)^2*cos(beta_t)^2*sin(alpha_t)^2 - Ip*M*d^2*m^2*cos(alpha_t)^2*cos(beta_t)^2 - Ip*M*d^2*m^2*sin(alpha_t)^2*sin(beta_t)^2))/(d^4*m^5*sin(alpha_t)^4 - Ip^2*m^3 - 3*Ip^2*M*m^2 - 3*Ip^2*M^2*m - d^4*m^5*sin(alpha_t)^2 - Ip^2*M^3 - Ip*d^2*m^4 + d^4*m^5*cos(beta_t)^2*sin(alpha_t)^2 - d^4*m^5*cos(beta_t)^2*sin(alpha_t)^4 + d^4*m^5*sin(alpha_t)^2*sin(beta_t)^2 - d^4*m^5*sin(alpha_t)^4*sin(beta_t)^2 - 3*M*d^4*m^4*sin(alpha_t)^2 + 2*M*d^4*m^4*sin(alpha_t)^4 - 3*Ip*M*d^2*m^3 - Ip*M^3*d^2*m - 3*M^2*d^4*m^3*sin(alpha_t)^2 - M^3*d^4*m^2*sin(alpha_t)^2 + M^2*d^4*m^3*sin(alpha_t)^4 - 3*Ip*M^2*d^2*m^2 + M^2*d^4*m^3*sin(alpha_t)^2*sin(beta_t)^2 - 2*Ip*M^2*d^2*m^2*sin(alpha_t)^2 + d^4*m^5*cos(alpha_t)^2*cos(beta_t)^2*sin(alpha_t)^2 - d^4*m^5*cos(alpha_t)^2*cos(beta_t)^4*sin(alpha_t)^2 + d^4*m^5*cos(alpha_t)^2*sin(alpha_t)^2*sin(beta_t)^2 - d^4*m^5*cos(alpha_t)^2*sin(alpha_t)^2*sin(beta_t)^4 + Ip*d^2*m^4*cos(alpha_t)^2*cos(beta_t)^2 + Ip*d^2*m^4*cos(alpha_t)^2*sin(beta_t)^2 + Ip*d^2*m^4*cos(beta_t)^2*sin(alpha_t)^2 + 2*M*d^4*m^4*cos(beta_t)^2*sin(alpha_t)^2 - M*d^4*m^4*cos(beta_t)^2*sin(alpha_t)^4 + Ip*d^2*m^4*sin(alpha_t)^2*sin(beta_t)^2 + 2*M*d^4*m^4*sin(alpha_t)^2*sin(beta_t)^2 - M*d^4*m^4*sin(alpha_t)^4*sin(beta_t)^2 - Ip*M*d^2*m^3*sin(alpha_t)^2 - Ip*M^3*d^2*m*sin(alpha_t)^2 + M^2*d^4*m^3*cos(beta_t)^2*sin(alpha_t)^2 + M^2*d^4*m^3*cos(alpha_t)^2*cos(beta_t)^2*sin(alpha_t)^2 + M^2*d^4*m^3*cos(alpha_t)^2*sin(alpha_t)^2*sin(beta_t)^2 + Ip*M^2*d^2*m^2*cos(alpha_t)^2*cos(beta_t)^2 + Ip*M^2*d^2*m^2*cos(alpha_t)^2*sin(beta_t)^2 + Ip*M^2*d^2*m^2*cos(beta_t)^2*sin(alpha_t)^2 + Ip*M^2*d^2*m^2*sin(alpha_t)^2*sin(beta_t)^2 - 2*d^4*m^5*cos(alpha_t)^2*cos(beta_t)^2*sin(alpha_t)^2*sin(beta_t)^2 + 2*M*d^4*m^4*cos(alpha_t)^2*cos(beta_t)^2*sin(alpha_t)^2 - M*d^4*m^4*cos(alpha_t)^2*cos(beta_t)^4*sin(alpha_t)^2 + 2*M*d^4*m^4*cos(alpha_t)^2*sin(alpha_t)^2*sin(beta_t)^2 - M*d^4*m^4*cos(alpha_t)^2*sin(alpha_t)^2*sin(beta_t)^4 + 2*Ip*M*d^2*m^3*cos(alpha_t)^2*cos(beta_t)^2 + 2*Ip*M*d^2*m^3*cos(alpha_t)^2*sin(beta_t)^2 + 2*Ip*M*d^2*m^3*cos(beta_t)^2*sin(alpha_t)^2 + 2*Ip*M*d^2*m^3*sin(alpha_t)^2*sin(beta_t)^2 - 2*M*d^4*m^4*cos(alpha_t)^2*cos(beta_t)^2*sin(alpha_t)^2*sin(beta_t)^2);
0, 0, 0, 0, 0, 0, 0, 0, 0, 0, 0,                                                                                                                                                                                                                                                                                                                                                                                                                                                                                                                                                                                                                                                                                                                                                                                                                                                                                                                                                                                                                                                                                                                                                                                                  0,                                                                                                                                                                                                                                                                                                                                                                                                                                                                                                                                                                                                                                                                                                                                                                                                                                                                                                                                                                                                                                                                                                                                                                                                                                                                                                                                                                                                                                                                  0,                                                                                                                                                                                                                                                                                                                                                                                                                                                                                                                                                                                                                                                                                                                                                                                                                                                                                                                                                                                                                                                                                                                                                                                                        0,                                                                                                                                                                                                                                                                                                                                                                                                                                                                                                                                                                                                                                                                                                                                                                                                                                                                                                                                                                                                                                                                                                                                                                                                                                                                                                                                                                                                                                                                                                                                                                                                                                                                                                                                                                                                                                                                                                                                                                                                                                                                                                                                                                                                                                                                                                                                                                                                                                                                                                                                                                                                                                                                                                                                                                                                                                                                                                                                                                                                                                                                                                                                                                                                                                                                                                                                                                                                                                                                                                                                                                                                                                                                                                                                                                                                                                                                                                                                                                                                                                                                                                                                                                                                                                                                                                                                                                                                                                                                                                                                                                                                                                                                                                                                                                                                                                                                                                                                                                                                                                                 (d^2*m^2*cos(alpha_t)*cos(beta_t)*sin(alpha_t)*(alpha_dot_t*d*m*cos(beta_t)*sin(alpha_t) + 2*beta_dot_t*d*m*cos(alpha_t)*sin(beta_t)))/(Ip*M^2 + Ip*m^2 + d^2*m^3 - d^2*m^3*sin(alpha_t)^2 + 2*M*d^2*m^2 + M^2*d^2*m + 2*Ip*M*m - d^2*m^3*cos(alpha_t)^2*cos(beta_t)^2 - d^2*m^3*cos(alpha_t)^2*sin(beta_t)^2 - M*d^2*m^2*sin(alpha_t)^2 - M*d^2*m^2*cos(alpha_t)^2*cos(beta_t)^2 - M*d^2*m^2*cos(alpha_t)^2*sin(beta_t)^2) - (alpha_dot_t*d*m*sin(alpha_t)*(d^2*m*cos(alpha_t)*cos(beta_t)^2*sin(alpha_t) - d^2*m*cos(alpha_t)*sin(alpha_t) + d^2*m*cos(alpha_t)*sin(alpha_t)*sin(beta_t)^2))/(- d^2*m^2*cos(alpha_t)^2*cos(beta_t)^2 - d^2*m^2*cos(alpha_t)^2*sin(beta_t)^2 - d^2*m^2*sin(alpha_t)^2 + d^2*m^2 + M*d^2*m + Ip*m + Ip*M) - (alpha_dot_t*d*m*cos(alpha_t)*(- d^2*m^2*cos(alpha_t)^2*cos(beta_t)^2 - d^2*m^2*cos(alpha_t)^2*sin(beta_t)^2 + d^2*m^2 + M*d^2*m + Ip*m + Ip*M))/(Ip*M^2 + Ip*m^2 + d^2*m^3 - d^2*m^3*sin(alpha_t)^2 + 2*M*d^2*m^2 + M^2*d^2*m + 2*Ip*M*m - d^2*m^3*cos(alpha_t)^2*cos(beta_t)^2 - d^2*m^3*cos(alpha_t)^2*sin(beta_t)^2 - M*d^2*m^2*sin(alpha_t)^2 - M*d^2*m^2*cos(alpha_t)^2*cos(beta_t)^2 - M*d^2*m^2*cos(alpha_t)^2*sin(beta_t)^2) - (d^2*m^2*cos(alpha_t)*sin(alpha_t)*sin(beta_t)*(2*beta_dot_t*d*m*cos(alpha_t)*cos(beta_t) - alpha_dot_t*d*m*sin(alpha_t)*sin(beta_t)))/(Ip*M^2 + Ip*m^2 + d^2*m^3 - d^2*m^3*sin(alpha_t)^2 + 2*M*d^2*m^2 + M^2*d^2*m + 2*Ip*M*m - d^2*m^3*cos(alpha_t)^2*cos(beta_t)^2 - d^2*m^3*cos(alpha_t)^2*sin(beta_t)^2 - M*d^2*m^2*sin(alpha_t)^2 - M*d^2*m^2*cos(alpha_t)^2*cos(beta_t)^2 - M*d^2*m^2*cos(alpha_t)^2*sin(beta_t)^2),                                                                                                                                                                                                                                                                                                                                                                                                                                                                                                                                                                                                                                                                                                                                                                                                                                                                                                                                                                                                                                                                                                                                                                                                                                                                                                                                                                                                                                                                                                                                                                                                                                                                                                                                                                                                                                                                                                                                                                                                                                                                                                                                                                                                                                                                                                                                                                                                                                                                                                                                                                                                                                                                                                                                                                                                                                                                                                                                                                                                                                                                                                                                                                                                                                                                                                                                                                                                                                                                                                                                                                                                                                                                                                                                                                                                                                                                                                                                                                                                                                                                                                                                                                                                                                                                                                                                                                                                                                                                                                                                                                                                                                                                                                                                                                                                                                                                                        (beta_dot_t*d^3*m^3*cos(alpha_t)*sin(alpha_t)^2*sin(beta_t)^2)/(Ip*M^2 + Ip*m^2 + d^2*m^3 - d^2*m^3*sin(alpha_t)^2 + 2*M*d^2*m^2 + M^2*d^2*m + 2*Ip*M*m - d^2*m^3*cos(alpha_t)^2*cos(beta_t)^2 - d^2*m^3*cos(alpha_t)^2*sin(beta_t)^2 - M*d^2*m^2*sin(alpha_t)^2 - M*d^2*m^2*cos(alpha_t)^2*cos(beta_t)^2 - M*d^2*m^2*cos(alpha_t)^2*sin(beta_t)^2) - (beta_dot_t*d*m*sin(alpha_t)*(m*cos(alpha_t)*sin(alpha_t)*d^2*cos(beta_t)^2 + m*cos(alpha_t)*sin(alpha_t)*d^2*sin(beta_t)^2))/(- d^2*m^2*cos(alpha_t)^2*cos(beta_t)^2 - d^2*m^2*cos(alpha_t)^2*sin(beta_t)^2 - d^2*m^2*sin(alpha_t)^2 + d^2*m^2 + M*d^2*m + Ip*m + Ip*M) + (beta_dot_t*d^3*m^3*cos(alpha_t)*cos(beta_t)^2*sin(alpha_t)^2)/(Ip*M^2 + Ip*m^2 + d^2*m^3 - d^2*m^3*sin(alpha_t)^2 + 2*M*d^2*m^2 + M^2*d^2*m + 2*Ip*M*m - d^2*m^3*cos(alpha_t)^2*cos(beta_t)^2 - d^2*m^3*cos(alpha_t)^2*sin(beta_t)^2 - M*d^2*m^2*sin(alpha_t)^2 - M*d^2*m^2*cos(alpha_t)^2*cos(beta_t)^2 - M*d^2*m^2*cos(alpha_t)^2*sin(beta_t)^2);
0, 0, 0, 0, 0, 0, 0, 0, 0, 0, 0, ((Iyy*cos(phi_t)*sin(phi_t)*sin(theta_t) - Izz*cos(phi_t)*sin(phi_t)*sin(theta_t))*(psi_dot_t*(Ixx*cos(theta_t) + Iyy*cos(phi_t)^2*cos(theta_t) - Izz*cos(phi_t)^2*cos(theta_t) - Iyy*cos(theta_t)*sin(phi_t)^2 + Izz*cos(theta_t)*sin(phi_t)^2) - theta_dot_t*(2*Iyy*cos(phi_t)*sin(phi_t) - 2*Izz*cos(phi_t)*sin(phi_t))))/(- cos(theta_t)*Iyy^2*cos(phi_t)^2*sin(phi_t)^2 - cos(theta_t)*Iyy^2*sin(phi_t)^4 + cos(theta_t)*Iyy^2*sin(phi_t)^2 + Izz*cos(theta_t)*Iyy*cos(phi_t)^2*sin(phi_t)^2 + Izz*cos(theta_t)*Iyy*cos(phi_t)^2 + Izz*cos(theta_t)*Iyy*sin(phi_t)^4) - ((psi_dot_t*(2*Iyy*cos(phi_t)*cos(theta_t)^2*sin(phi_t) - 2*Izz*cos(phi_t)*cos(theta_t)^2*sin(phi_t)) - theta_dot_t*(Ixx*cos(theta_t) - Iyy*cos(phi_t)^2*cos(theta_t) + Izz*cos(phi_t)^2*cos(theta_t) + Iyy*cos(theta_t)*sin(phi_t)^2 - Izz*cos(theta_t)*sin(phi_t)^2))*(Iyy*sin(theta_t) - Iyy*sin(phi_t)^2*sin(theta_t) + Izz*sin(phi_t)^2*sin(theta_t)))/(- Iyy^2*cos(phi_t)^2*cos(theta_t)^2*sin(phi_t)^2 - Iyy^2*cos(theta_t)^2*sin(phi_t)^4 + Iyy^2*cos(theta_t)^2*sin(phi_t)^2 + Izz*Iyy*cos(phi_t)^2*cos(theta_t)^2*sin(phi_t)^2 + Izz*Iyy*cos(phi_t)^2*cos(theta_t)^2 + Izz*Iyy*cos(theta_t)^2*sin(phi_t)^4), ((theta_dot_t*(Iyy*cos(phi_t)*sin(phi_t)*sin(theta_t) - Izz*cos(phi_t)*sin(phi_t)*sin(theta_t)) + psi_dot_t*(2*Izz*cos(phi_t)^2*cos(theta_t)*sin(theta_t) - 2*Ixx*cos(theta_t)*sin(theta_t) + 2*Iyy*cos(theta_t)*sin(phi_t)^2*sin(theta_t)))*(Iyy*sin(theta_t) - Iyy*sin(phi_t)^2*sin(theta_t) + Izz*sin(phi_t)^2*sin(theta_t)))/(- Iyy^2*cos(phi_t)^2*cos(theta_t)^2*sin(phi_t)^2 - Iyy^2*cos(theta_t)^2*sin(phi_t)^4 + Iyy^2*cos(theta_t)^2*sin(phi_t)^2 + Izz*Iyy*cos(phi_t)^2*cos(theta_t)^2*sin(phi_t)^2 + Izz*Iyy*cos(phi_t)^2*cos(theta_t)^2 + Izz*Iyy*cos(theta_t)^2*sin(phi_t)^4) + ((psi_dot_t*(Ixx*cos(theta_t) + Iyy*cos(phi_t)^2*cos(theta_t) - Izz*cos(phi_t)^2*cos(theta_t) - Iyy*cos(theta_t)*sin(phi_t)^2 + Izz*cos(theta_t)*sin(phi_t)^2) - theta_dot_t*(Iyy*cos(phi_t)*sin(phi_t) - Izz*cos(phi_t)*sin(phi_t)))*(- Iyy^2*cos(phi_t)^2*cos(theta_t)^2*sin(phi_t)^2 - Iyy^2*cos(theta_t)^2*sin(phi_t)^4 + Iyy^2*cos(theta_t)^2*sin(phi_t)^2 + Izz*Iyy*cos(phi_t)^2*cos(theta_t)^2*sin(phi_t)^2 + Izz*Iyy*cos(phi_t)^2*cos(theta_t)^2 + Izz*Iyy*cos(theta_t)^2*sin(phi_t)^4 - Ixx*Iyy*sin(phi_t)^2*sin(theta_t)^2 + Ixx*Iyy*sin(theta_t)^2 + Ixx*Izz*sin(phi_t)^2*sin(theta_t)^2))/(Ixx*(- Iyy^2*cos(phi_t)^2*cos(theta_t)^2*sin(phi_t)^2 - Iyy^2*cos(theta_t)^2*sin(phi_t)^4 + Iyy^2*cos(theta_t)^2*sin(phi_t)^2 + Izz*Iyy*cos(phi_t)^2*cos(theta_t)^2*sin(phi_t)^2 + Izz*Iyy*cos(phi_t)^2*cos(theta_t)^2 + Izz*Iyy*cos(theta_t)^2*sin(phi_t)^4)), (psi_dot_t*(Iyy*cos(phi_t)*sin(phi_t)*sin(theta_t) - Izz*cos(phi_t)*sin(phi_t)*sin(theta_t))*(Izz*cos(phi_t)^2*cos(theta_t)*sin(theta_t) - Ixx*cos(theta_t)*sin(theta_t) + Iyy*cos(theta_t)*sin(phi_t)^2*sin(theta_t)))/(- cos(theta_t)*Iyy^2*cos(phi_t)^2*sin(phi_t)^2 - cos(theta_t)*Iyy^2*sin(phi_t)^4 + cos(theta_t)*Iyy^2*sin(phi_t)^2 + Izz*cos(theta_t)*Iyy*cos(phi_t)^2*sin(phi_t)^2 + Izz*cos(theta_t)*Iyy*cos(phi_t)^2 + Izz*cos(theta_t)*Iyy*sin(phi_t)^4) + (psi_dot_t*(Iyy*cos(phi_t)*cos(theta_t)^2*sin(phi_t) - Izz*cos(phi_t)*cos(theta_t)^2*sin(phi_t))*(- Iyy^2*cos(phi_t)^2*cos(theta_t)^2*sin(phi_t)^2 - Iyy^2*cos(theta_t)^2*sin(phi_t)^4 + Iyy^2*cos(theta_t)^2*sin(phi_t)^2 + Izz*Iyy*cos(phi_t)^2*cos(theta_t)^2*sin(phi_t)^2 + Izz*Iyy*cos(phi_t)^2*cos(theta_t)^2 + Izz*Iyy*cos(theta_t)^2*sin(phi_t)^4 - Ixx*Iyy*sin(phi_t)^2*sin(theta_t)^2 + Ixx*Iyy*sin(theta_t)^2 + Ixx*Izz*sin(phi_t)^2*sin(theta_t)^2))/(Ixx*(- Iyy^2*cos(phi_t)^2*cos(theta_t)^2*sin(phi_t)^2 - Iyy^2*cos(theta_t)^2*sin(phi_t)^4 + Iyy^2*cos(theta_t)^2*sin(phi_t)^2 + Izz*Iyy*cos(phi_t)^2*cos(theta_t)^2*sin(phi_t)^2 + Izz*Iyy*cos(phi_t)^2*cos(theta_t)^2 + Izz*Iyy*cos(theta_t)^2*sin(phi_t)^4)),                                                                                                                                                                                                                                                                                                                                                                                                                                                                                                                                                                                                                                                                                                                                                                                                                                                                                                                                                                                                                                                                                                                                                                                                                                                                                                                                                                                                                                                                                                                                                                                                                                                                                                                                                                                                                                                                                                                                                                                                                                                                                                                                                                                                                                                                                                                                                                                                                                                                                                                                                                                                                                                                                                                                                                                                                                                                                                                                                                                                                                                                                                                                                                                                                                                                                                                                                                                                                                                                                                                                                                                                                                                                                                                                                                                                                                                                                                                                                                                                                                                                                                                                                                                                                                                                                                                                                                                                                                                                                                                                                                                                                                                                                                                                                                                                                                                                                                                                                                                                                                                                                                                                                                                                                                                                                                                                                                                                                                                                                                                                                                                                                                                                                                                                                                                                                                                                                                                                                                                                                                                                                                                                                                                                                                                                                                                                                                                                                                                                                                                                                                                                                                                               0,                                                                                                                                                                                                                                                                                                                                                                                                                                                                                                                                                                                                                                                                                                                                                                                                                                                                                                                                                                                                                                                                                                                                                                                                                                                                                                                                                                                                                                                                                                                                                                                                                                                                                                                                                                                                                                                                                                                                                                                                                                                                                                                                                                                                                                                                                                                                                                                                                                                                                                                                                                                                                                                                                                                                                                                                                                                                                                                                                                                                                                                                                                                                                                                                                                                                                                                                                                                                                                                                                                                                                                                                                                                                                                                                                                                                                                                                                                                                                                                                                                                                                                                                                                                                                                                                                                                                                                                                                                                                                                                                                                                                                                                                                                                                                                                                                                                                                                                                                                                                                                                                                                                                                                                                                                                                                                                                                                                                                                                                                                                                                                                                                                                                                                                                                                                                                                                                           0;
0, 0, 0, 0, 0, 0, 0, 0, 0, 0, 0,                                                                                                                                                                  ((Iyy*cos(phi_t)*sin(phi_t) - Izz*cos(phi_t)*sin(phi_t))*(psi_dot_t*(2*Iyy*cos(phi_t)*cos(theta_t)^2*sin(phi_t) - 2*Izz*cos(phi_t)*cos(theta_t)^2*sin(phi_t)) - theta_dot_t*(Ixx*cos(theta_t) - Iyy*cos(phi_t)^2*cos(theta_t) + Izz*cos(phi_t)^2*cos(theta_t) + Iyy*cos(theta_t)*sin(phi_t)^2 - Izz*cos(theta_t)*sin(phi_t)^2)))/(- cos(theta_t)*Iyy^2*cos(phi_t)^2*sin(phi_t)^2 - cos(theta_t)*Iyy^2*sin(phi_t)^4 + cos(theta_t)*Iyy^2*sin(phi_t)^2 + Izz*cos(theta_t)*Iyy*cos(phi_t)^2*sin(phi_t)^2 + Izz*cos(theta_t)*Iyy*cos(phi_t)^2 + Izz*cos(theta_t)*Iyy*sin(phi_t)^4) - ((Izz*cos(phi_t)^2 + Iyy*sin(phi_t)^2)*(psi_dot_t*(Ixx*cos(theta_t) + Iyy*cos(phi_t)^2*cos(theta_t) - Izz*cos(phi_t)^2*cos(theta_t) - Iyy*cos(theta_t)*sin(phi_t)^2 + Izz*cos(theta_t)*sin(phi_t)^2) - theta_dot_t*(2*Iyy*cos(phi_t)*sin(phi_t) - 2*Izz*cos(phi_t)*sin(phi_t))))/(- Iyy^2*cos(phi_t)^2*sin(phi_t)^2 - Iyy^2*sin(phi_t)^4 + Iyy^2*sin(phi_t)^2 + Izz*Iyy*cos(phi_t)^2*sin(phi_t)^2 + Izz*Iyy*cos(phi_t)^2 + Izz*Iyy*sin(phi_t)^4),                                                                                                                                                                                                                                                                                                                                     - ((theta_dot_t*(Iyy*cos(phi_t)*sin(phi_t)*sin(theta_t) - Izz*cos(phi_t)*sin(phi_t)*sin(theta_t)) + psi_dot_t*(2*Izz*cos(phi_t)^2*cos(theta_t)*sin(theta_t) - 2*Ixx*cos(theta_t)*sin(theta_t) + 2*Iyy*cos(theta_t)*sin(phi_t)^2*sin(theta_t)))*(Iyy*cos(phi_t)*sin(phi_t) - Izz*cos(phi_t)*sin(phi_t)))/(- cos(theta_t)*Iyy^2*cos(phi_t)^2*sin(phi_t)^2 - cos(theta_t)*Iyy^2*sin(phi_t)^4 + cos(theta_t)*Iyy^2*sin(phi_t)^2 + Izz*cos(theta_t)*Iyy*cos(phi_t)^2*sin(phi_t)^2 + Izz*cos(theta_t)*Iyy*cos(phi_t)^2 + Izz*cos(theta_t)*Iyy*sin(phi_t)^4) - ((Iyy*cos(phi_t)*sin(phi_t)*sin(theta_t) - Izz*cos(phi_t)*sin(phi_t)*sin(theta_t))*(psi_dot_t*(Ixx*cos(theta_t) + Iyy*cos(phi_t)^2*cos(theta_t) - Izz*cos(phi_t)^2*cos(theta_t) - Iyy*cos(theta_t)*sin(phi_t)^2 + Izz*cos(theta_t)*sin(phi_t)^2) - theta_dot_t*(Iyy*cos(phi_t)*sin(phi_t) - Izz*cos(phi_t)*sin(phi_t))))/(- cos(theta_t)*Iyy^2*cos(phi_t)^2*sin(phi_t)^2 - cos(theta_t)*Iyy^2*sin(phi_t)^4 + cos(theta_t)*Iyy^2*sin(phi_t)^2 + Izz*cos(theta_t)*Iyy*cos(phi_t)^2*sin(phi_t)^2 + Izz*cos(theta_t)*Iyy*cos(phi_t)^2 + Izz*cos(theta_t)*Iyy*sin(phi_t)^4),                                                                                                                                                                                                                                                                                                                                                                                                                        - (psi_dot_t*(Izz*cos(phi_t)^2 + Iyy*sin(phi_t)^2)*(Izz*cos(phi_t)^2*cos(theta_t)*sin(theta_t) - Ixx*cos(theta_t)*sin(theta_t) + Iyy*cos(theta_t)*sin(phi_t)^2*sin(theta_t)))/(- Iyy^2*cos(phi_t)^2*sin(phi_t)^2 - Iyy^2*sin(phi_t)^4 + Iyy^2*sin(phi_t)^2 + Izz*Iyy*cos(phi_t)^2*sin(phi_t)^2 + Izz*Iyy*cos(phi_t)^2 + Izz*Iyy*sin(phi_t)^4) - (psi_dot_t*(Iyy*cos(phi_t)*cos(theta_t)^2*sin(phi_t) - Izz*cos(phi_t)*cos(theta_t)^2*sin(phi_t))*(Iyy*cos(phi_t)*sin(phi_t)*sin(theta_t) - Izz*cos(phi_t)*sin(phi_t)*sin(theta_t)))/(- cos(theta_t)*Iyy^2*cos(phi_t)^2*sin(phi_t)^2 - cos(theta_t)*Iyy^2*sin(phi_t)^4 + cos(theta_t)*Iyy^2*sin(phi_t)^2 + Izz*cos(theta_t)*Iyy*cos(phi_t)^2*sin(phi_t)^2 + Izz*cos(theta_t)*Iyy*cos(phi_t)^2 + Izz*cos(theta_t)*Iyy*sin(phi_t)^4),                                                                                                                                                                                                                                                                                                                                                                                                                                                                                                                                                                                                                                                                                                                                                                                                                                                                                                                                                                                                                                                                                                                                                                                                                                                                                                                                                                                                                                                                                                                                                                                                                                                                                                                                                                                                                                                                                                                                                                                                                                                                                                                                                                                                                                                                                                                                                                                                                                                                                                                                                                                                                                                                                                                                                                                                                                                                                                                                                                                                                                                                                                                                                                                                                                                                                                                                                                                                                                                                                                                                                                                                                                                                                                                                                                                                                                                                                                                                                                                                                                                                                                                                                                                                                                                                                                                                                                                                                                                                                                                                                                                                                                                                                                                                                                                                                                                                                                                                                                                                                                                                                                                                                                                                                                                                                                                                                                                                                                                                                                                                                                                                                                                                                                                                                                                                                                                                                                                                                                                                                                                                                                                                                                                                                                                                                                                                                                                                                                                                                                                                                                                                                                                               0,                                                                                                                                                                                                                                                                                                                                                                                                                                                                                                                                                                                                                                                                                                                                                                                                                                                                                                                                                                                                                                                                                                                                                                                                                                                                                                                                                                                                                                                                                                                                                                                                                                                                                                                                                                                                                                                                                                                                                                                                                                                                                                                                                                                                                                                                                                                                                                                                                                                                                                                                                                                                                                                                                                                                                                                                                                                                                                                                                                                                                                                                                                                                                                                                                                                                                                                                                                                                                                                                                                                                                                                                                                                                                                                                                                                                                                                                                                                                                                                                                                                                                                                                                                                                                                                                                                                                                                                                                                                                                                                                                                                                                                                                                                                                                                                                                                                                                                                                                                                                                                                                                                                                                                                                                                                                                                                                                                                                                                                                                                                                                                                                                                                                                                                                                                                                                                                                           0;
0, 0, 0, 0, 0, 0, 0, 0, 0, 0, 0,                                                                  ((Iyy*cos(phi_t)*sin(phi_t) - Izz*cos(phi_t)*sin(phi_t))*(psi_dot_t*(Ixx*cos(theta_t) + Iyy*cos(phi_t)^2*cos(theta_t) - Izz*cos(phi_t)^2*cos(theta_t) - Iyy*cos(theta_t)*sin(phi_t)^2 + Izz*cos(theta_t)*sin(phi_t)^2) - theta_dot_t*(2*Iyy*cos(phi_t)*sin(phi_t) - 2*Izz*cos(phi_t)*sin(phi_t))))/(- cos(theta_t)*Iyy^2*cos(phi_t)^2*sin(phi_t)^2 - cos(theta_t)*Iyy^2*sin(phi_t)^4 + cos(theta_t)*Iyy^2*sin(phi_t)^2 + Izz*cos(theta_t)*Iyy*cos(phi_t)^2*sin(phi_t)^2 + Izz*cos(theta_t)*Iyy*cos(phi_t)^2 + Izz*cos(theta_t)*Iyy*sin(phi_t)^4) - ((psi_dot_t*(2*Iyy*cos(phi_t)*cos(theta_t)^2*sin(phi_t) - 2*Izz*cos(phi_t)*cos(theta_t)^2*sin(phi_t)) - theta_dot_t*(Ixx*cos(theta_t) - Iyy*cos(phi_t)^2*cos(theta_t) + Izz*cos(phi_t)^2*cos(theta_t) + Iyy*cos(theta_t)*sin(phi_t)^2 - Izz*cos(theta_t)*sin(phi_t)^2))*(Iyy - Iyy*sin(phi_t)^2 + Izz*sin(phi_t)^2))/(- Iyy^2*cos(phi_t)^2*cos(theta_t)^2*sin(phi_t)^2 - Iyy^2*cos(theta_t)^2*sin(phi_t)^4 + Iyy^2*cos(theta_t)^2*sin(phi_t)^2 + Izz*Iyy*cos(phi_t)^2*cos(theta_t)^2*sin(phi_t)^2 + Izz*Iyy*cos(phi_t)^2*cos(theta_t)^2 + Izz*Iyy*cos(theta_t)^2*sin(phi_t)^4),                                                                                                                                                                                                                                                                                                                          ((theta_dot_t*(Iyy*cos(phi_t)*sin(phi_t)*sin(theta_t) - Izz*cos(phi_t)*sin(phi_t)*sin(theta_t)) + psi_dot_t*(2*Izz*cos(phi_t)^2*cos(theta_t)*sin(theta_t) - 2*Ixx*cos(theta_t)*sin(theta_t) + 2*Iyy*cos(theta_t)*sin(phi_t)^2*sin(theta_t)))*(Iyy - Iyy*sin(phi_t)^2 + Izz*sin(phi_t)^2))/(- Iyy^2*cos(phi_t)^2*cos(theta_t)^2*sin(phi_t)^2 - Iyy^2*cos(theta_t)^2*sin(phi_t)^4 + Iyy^2*cos(theta_t)^2*sin(phi_t)^2 + Izz*Iyy*cos(phi_t)^2*cos(theta_t)^2*sin(phi_t)^2 + Izz*Iyy*cos(phi_t)^2*cos(theta_t)^2 + Izz*Iyy*cos(theta_t)^2*sin(phi_t)^4) + ((psi_dot_t*(Ixx*cos(theta_t) + Iyy*cos(phi_t)^2*cos(theta_t) - Izz*cos(phi_t)^2*cos(theta_t) - Iyy*cos(theta_t)*sin(phi_t)^2 + Izz*cos(theta_t)*sin(phi_t)^2) - theta_dot_t*(Iyy*cos(phi_t)*sin(phi_t) - Izz*cos(phi_t)*sin(phi_t)))*(Iyy*sin(theta_t) - Iyy*sin(phi_t)^2*sin(theta_t) + Izz*sin(phi_t)^2*sin(theta_t)))/(- Iyy^2*cos(phi_t)^2*cos(theta_t)^2*sin(phi_t)^2 - Iyy^2*cos(theta_t)^2*sin(phi_t)^4 + Iyy^2*cos(theta_t)^2*sin(phi_t)^2 + Izz*Iyy*cos(phi_t)^2*cos(theta_t)^2*sin(phi_t)^2 + Izz*Iyy*cos(phi_t)^2*cos(theta_t)^2 + Izz*Iyy*cos(theta_t)^2*sin(phi_t)^4),                                                                                                                                                                                                                                                                                                             (psi_dot_t*(Iyy*cos(phi_t)*sin(phi_t) - Izz*cos(phi_t)*sin(phi_t))*(Izz*cos(phi_t)^2*cos(theta_t)*sin(theta_t) - Ixx*cos(theta_t)*sin(theta_t) + Iyy*cos(theta_t)*sin(phi_t)^2*sin(theta_t)))/(- cos(theta_t)*Iyy^2*cos(phi_t)^2*sin(phi_t)^2 - cos(theta_t)*Iyy^2*sin(phi_t)^4 + cos(theta_t)*Iyy^2*sin(phi_t)^2 + Izz*cos(theta_t)*Iyy*cos(phi_t)^2*sin(phi_t)^2 + Izz*cos(theta_t)*Iyy*cos(phi_t)^2 + Izz*cos(theta_t)*Iyy*sin(phi_t)^4) + (psi_dot_t*(Iyy*cos(phi_t)*cos(theta_t)^2*sin(phi_t) - Izz*cos(phi_t)*cos(theta_t)^2*sin(phi_t))*(Iyy*sin(theta_t) - Iyy*sin(phi_t)^2*sin(theta_t) + Izz*sin(phi_t)^2*sin(theta_t)))/(- Iyy^2*cos(phi_t)^2*cos(theta_t)^2*sin(phi_t)^2 - Iyy^2*cos(theta_t)^2*sin(phi_t)^4 + Iyy^2*cos(theta_t)^2*sin(phi_t)^2 + Izz*Iyy*cos(phi_t)^2*cos(theta_t)^2*sin(phi_t)^2 + Izz*Iyy*cos(phi_t)^2*cos(theta_t)^2 + Izz*Iyy*cos(theta_t)^2*sin(phi_t)^4),                                                                                                                                                                                                                                                                                                                                                                                                                                                                                                                                                                                                                                                                                                                                                                                                                                                                                                                                                                                                                                                                                                                                                                                                                                                                                                                                                                                                                                                                                                                                                                                                                                                                                                                                                                                                                                                                                                                                                                                                                                                                                                                                                                                                                                                                                                                                                                                                                                                                                                                                                                                                                                                                                                                                                                                                                                                                                                                                                                                                                                                                                                                                                                                                                                                                                                                                                                                                                                                                                                                                                                                                                                                                                                                                                                                                                                                                                                                                                                                                                                                                                                                                                                                                                                                                                                                                                                                                                                                                                                                                                                                                                                                                                                                                                                                                                                                                                                                                                                                                                                                                                                                                                                                                                                                                                                                                                                                                                                                                                                                                                                                                                                                                                                                                                                                                                                                                                                                                                                                                                                                                                                                                                                                                                                                                                                                                                                                                                                                                                                                                                                                                                                                               0,                                                                                                                                                                                                                                                                                                                                                                                                                                                                                                                                                                                                                                                                                                                                                                                                                                                                                                                                                                                                                                                                                                                                                                                                                                                                                                                                                                                                                                                                                                                                                                                                                                                                                                                                                                                                                                                                                                                                                                                                                                                                                                                                                                                                                                                                                                                                                                                                                                                                                                                                                                                                                                                                                                                                                                                                                                                                                                                                                                                                                                                                                                                                                                                                                                                                                                                                                                                                                                                                                                                                                                                                                                                                                                                                                                                                                                                                                                                                                                                                                                                                                                                                                                                                                                                                                                                                                                                                                                                                                                                                                                                                                                                                                                                                                                                                                                                                                                                                                                                                                                                                                                                                                                                                                                                                                                                                                                                                                                                                                                                                                                                                                                                                                                                                                                                                                                                                           0;
0, 0, 0, 0, 0, 0, 0, 0, 0, 0, 0,                                                                                                                                                                                                                                                                                                                                                                                                                                                                                                                                                                                                                                                                                                                                                                                                                                                                                                                                                                                                                                                                                                                                                                                                  0,                                                                                                                                                                                                                                                                                                                                                                                                                                                                                                                                                                                                                                                                                                                                                                                                                                                                                                                                                                                                                                                                                                                                                                                                                                                                                                                                                                                                                                                                  0,                                                                                                                                                                                                                                                                                                                                                                                                                                                                                                                                                                                                                                                                                                                                                                                                                                                                                                                                                                                                                                                                                                                                                                                                        0,                                                                                                                                                                                                                                                                                                                                                                                                                                                                                                                                                                                                                                                                                                                                                                                                                                                                                                                                                                                                                                                                                                                                                                                                                                                                                                                                                                                                                                                                                                                                                                                                                                                                                                                                                                                                                                                                                                                                                                                                                                                                                                                                                                                                                                                                                                                                                                                                                                                                                                                                                                                                                                                                                                                                                                                                                                                                                                                                                                                                                                                                                                                                                                                                                                                                                                                                                                                                                                                                                                                                                                                                                                                                                                                                                                                                                                                                                                                                                                                                                                                                                                                                                                                                                                                                                                                                                                                                                                                                                                                                                                                                                                                                                                                                                                                                                                                                                                                                                                                                                                                                                                                                                                                                                                                                                                                                                                                                                                                                                                                                                                                                                           (alpha_dot_t*(M + m)*(d^2*m*cos(alpha_t)*cos(beta_t)^2*sin(alpha_t) - d^2*m*cos(alpha_t)*sin(alpha_t) + d^2*m*cos(alpha_t)*sin(alpha_t)*sin(beta_t)^2))/(- d^2*m^2*cos(alpha_t)^2*cos(beta_t)^2 - d^2*m^2*cos(alpha_t)^2*sin(beta_t)^2 - d^2*m^2*sin(alpha_t)^2 + d^2*m^2 + M*d^2*m + Ip*m + Ip*M) + (alpha_dot_t*d^2*m^2*cos(alpha_t)*sin(alpha_t))/(- d^2*m^2*cos(alpha_t)^2*cos(beta_t)^2 - d^2*m^2*cos(alpha_t)^2*sin(beta_t)^2 - d^2*m^2*sin(alpha_t)^2 + d^2*m^2 + M*d^2*m + Ip*m + Ip*M) - (d*m*cos(alpha_t)*cos(beta_t)*(alpha_dot_t*d*m*cos(beta_t)*sin(alpha_t) + 2*beta_dot_t*d*m*cos(alpha_t)*sin(beta_t)))/(- d^2*m^2*cos(alpha_t)^2*cos(beta_t)^2 - d^2*m^2*cos(alpha_t)^2*sin(beta_t)^2 - d^2*m^2*sin(alpha_t)^2 + d^2*m^2 + M*d^2*m + Ip*m + Ip*M) + (d*m*cos(alpha_t)*sin(beta_t)*(2*beta_dot_t*d*m*cos(alpha_t)*cos(beta_t) - alpha_dot_t*d*m*sin(alpha_t)*sin(beta_t)))/(- d^2*m^2*cos(alpha_t)^2*cos(beta_t)^2 - d^2*m^2*cos(alpha_t)^2*sin(beta_t)^2 - d^2*m^2*sin(alpha_t)^2 + d^2*m^2 + M*d^2*m + Ip*m + Ip*M),                                                                                                                                                                                                                                                                                                                                                                                                                                                                                                                                                                                                                                                                                                                                                                                                                                                                                                                                                                                                                                                                                                                                                                                                                                                                                                                                                                                                                                                                                                                                                                                                                                                                                                                                                                                                                                                                                                                                                                                                                                                                                                                                                                                                                                                                                                                                                                                                                                                                                                                                                                                                                                                                                                                                                                                                                                                                                                                                                                                                                                                                                                                                                                                                                                                                                                                                                                                                                                                                                                                                                                                                                                                                                                                                                                                                                                                                                                                                                                                                                                                                                                                                                                                                                                                                                                                                                                                                                                                                                                                                                                                                                                                                                                                                                                                                                                                                                                                                                                                                                                                                                                                                                                                         (beta_dot_t*(m*cos(alpha_t)*sin(alpha_t)*d^2*cos(beta_t)^2 + m*cos(alpha_t)*sin(alpha_t)*d^2*sin(beta_t)^2)*(M + m))/(- d^2*m^2*cos(alpha_t)^2*cos(beta_t)^2 - d^2*m^2*cos(alpha_t)^2*sin(beta_t)^2 - d^2*m^2*sin(alpha_t)^2 + d^2*m^2 + M*d^2*m + Ip*m + Ip*M) - (beta_dot_t*d^2*m^2*cos(alpha_t)*cos(beta_t)^2*sin(alpha_t))/(- d^2*m^2*cos(alpha_t)^2*cos(beta_t)^2 - d^2*m^2*cos(alpha_t)^2*sin(beta_t)^2 - d^2*m^2*sin(alpha_t)^2 + d^2*m^2 + M*d^2*m + Ip*m + Ip*M) - (beta_dot_t*d^2*m^2*cos(alpha_t)*sin(alpha_t)*sin(beta_t)^2)/(- d^2*m^2*cos(alpha_t)^2*cos(beta_t)^2 - d^2*m^2*cos(alpha_t)^2*sin(beta_t)^2 - d^2*m^2*sin(alpha_t)^2 + d^2*m^2 + M*d^2*m + Ip*m + Ip*M);
0, 0, 0, 0, 0, 0, 0, 0, 0, 0, 0,                                                                                                                                                                                                                                                                                                                                                                                                                                                                                                                                                                                                                                                                                                                                                                                                                                                                                                                                                                                                                                                                                                                                                                                                  0,                                                                                                                                                                                                                                                                                                                                                                                                                                                                                                                                                                                                                                                                                                                                                                                                                                                                                                                                                                                                                                                                                                                                                                                                                                                                                                                                                                                                                                                                  0,                                                                                                                                                                                                                                                                                                                                                                                                                                                                                                                                                                                                                                                                                                                                                                                                                                                                                                                                                                                                                                                                                                                                                                                                        0,                                                                                                                                                                                                                                                                                                                                                                                                                                                                                                                                                                                                                                                                                                                                                                                                                                                                                                                                                                                                                                                                                                                                                                                                                                                                                                                                                                                                                                                                                                                                                                                                                                                                                                                                                                                                                                                                                                                                                                                                                                                                                                                                                                                                                                                                                                                                                                                                                                                                                                                                                                                                                                                                                                                                                                                                                                                                                                                                                                                                                                                                                                                                                                                                                                                                                                                                                                                                                                                                                                                                                                                                                                                                                                                                                                                                                                                                                                                                                                                                                                                                                                                                                                                                                                                                                                                                                                                                                                                                                                                                                                                                                                                                                                                                                                                                                                                                                                                                                                                                                                                                                                                                                                                                                                                                                                                                                                                                                                                                                                                                                                                                                                                                                                                                                                                                                                        (d*m*cos(beta_t)*sin(alpha_t)*(2*beta_dot_t*d*m*cos(alpha_t)*cos(beta_t) - alpha_dot_t*d*m*sin(alpha_t)*sin(beta_t)))/(- d^2*m^2*cos(beta_t)^2*sin(alpha_t)^2 - d^2*m^2*sin(alpha_t)^2*sin(beta_t)^2 + d^2*m^2*sin(alpha_t)^2 + M*d^2*m*sin(alpha_t)^2 + Ip*m + Ip*M) - (beta_dot_t*(2*d^2*m*cos(alpha_t)*cos(beta_t)^2*sin(alpha_t) + 2*d^2*m*cos(alpha_t)*sin(alpha_t)*sin(beta_t)^2)*(M + m))/(- d^2*m^2*cos(beta_t)^2*sin(alpha_t)^2 - d^2*m^2*sin(alpha_t)^2*sin(beta_t)^2 + d^2*m^2*sin(alpha_t)^2 + M*d^2*m*sin(alpha_t)^2 + Ip*m + Ip*M) + (d*m*sin(alpha_t)*sin(beta_t)*(alpha_dot_t*d*m*cos(beta_t)*sin(alpha_t) + 2*beta_dot_t*d*m*cos(alpha_t)*sin(beta_t)))/(- d^2*m^2*cos(beta_t)^2*sin(alpha_t)^2 - d^2*m^2*sin(alpha_t)^2*sin(beta_t)^2 + d^2*m^2*sin(alpha_t)^2 + M*d^2*m*sin(alpha_t)^2 + Ip*m + Ip*M),                                                                                                                                                                                                                                                                                                                                                                                                                                                                                                                                                                                                                                                                                                                                                                                                                                                                                                                                                                                                                                                                                                                                                                                                                                                                                                                                                                                                                                                                                                                                                                                                                                                                                                                                                                                                                                                                                                                                                                                                                                                                                                                                                                                                                                                                                                                                                                                                                                                                                                                                                                                                                                                                                                                                                                                                                                                                                                                                                                                                                                                                                                                                                                                                                                                                                                                                                                                                                                                                                                                                                                                                                                                                                                                                                                                                                                                                                                                                                                                                                                                                                                                                                                                                                                                                                                                                                                                                                                                                                                                                                                                                                                                                                                                                                                                                                                                                                                                                                                                                                                                                                                                                                                                                                                                                                                                                                                                                                                                                                                                                                                                                                                                                                                                                                                                                                                                                           0];
